simulink model "simsim"  (R2022b)
settings: Solver=VariableStepAuto  StartTime=0.0  StopTime=10.0  RelTol=1e-3
settings Model: Creator=zhanghanwen  LastModifiedBy=zhanghanwen

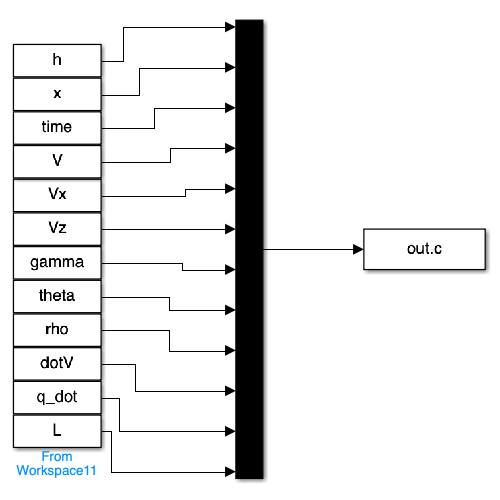
[thumbnail: Simulink's stored preview of the top-level diagram]
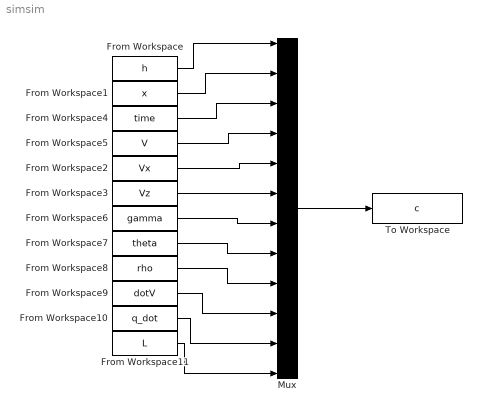
== system simsim ==
  From Workspace : FromWorkspace  VariableName=h
  From Workspace1 : FromWorkspace  VariableName=x
  From Workspace10 : FromWorkspace  VariableName=q_dot
  From Workspace11 : FromWorkspace  VariableName=L
  From Workspace2 : FromWorkspace  VariableName=Vx
  From Workspace3 : FromWorkspace  VariableName=Vz
  From Workspace4 : FromWorkspace  VariableName=time
  From Workspace5 : FromWorkspace  VariableName=V
  From Workspace6 : FromWorkspace  VariableName=gamma
  From Workspace7 : FromWorkspace  VariableName=theta
  From Workspace8 : FromWorkspace  VariableName=rho
  From Workspace9 : FromWorkspace  VariableName=dotV
  Mux : Mux  Inputs=12
  To Workspace : ToWorkspace  VariableName=c  SaveFormat=Timeseries  SampleTime=-1
  wires:
  From Workspace/1 -> Mux/1
  From Workspace1/1 -> Mux/2
  From Workspace4/1 -> Mux/3
  From Workspace5/1 -> Mux/4
  From Workspace2/1 -> Mux/5
  From Workspace3/1 -> Mux/6
  From Workspace6/1 -> Mux/7
  From Workspace7/1 -> Mux/8
  From Workspace8/1 -> Mux/9
  From Workspace9/1 -> Mux/10
  From Workspace10/1 -> Mux/11
  From Workspace11/1 -> Mux/12
  Mux/1 -> To Workspace/1
